simulink model "d5_a_1_model"  (R2025a)
settings: Solver=VariableStepAuto  StartTime=0.0  StopTime=10.0  RelTol=1e-3
undefined symbols (not defined in the file): A, B, Rk, Sk, Tsk
settings Model: Creator=Korisnik  LastModifiedBy=Korisnik

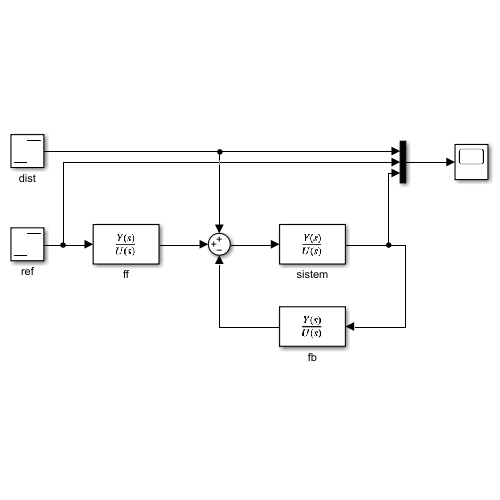
[thumbnail: Simulink's stored preview of the top-level diagram]
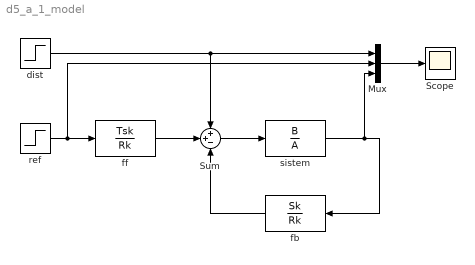
== system d5_a_1_model ==
  Mux : Mux  Inputs=3
  Scope : Scope
      settings: ActiveDisplayYMinimum=-1.2499999999999998  ActiveDisplayYMaximum=11.25
  Sum : Sum  Inputs=++-
  dist : Step  Time=5  After=10  SampleTime=0
  fb : TransferFcn  Numerator=Sk  Denominator=Rk
  ff : TransferFcn  Numerator=Tsk  Denominator=Rk
  ref : Step  Time=0  After=8  SampleTime=0
  sistem : TransferFcn  Numerator=B  Denominator=A
  wires:
  sistem/1 -> Mux/3, fb/1
  ff/1 -> Sum/2
  ref/1 -> Mux/2, ff/1
  fb/1 -> Sum/3
  Sum/1 -> sistem/1
  dist/1 -> Mux/1, Sum/1
  Mux/1 -> Scope/1
